simulink model "program_flight"  (R2022a)
settings: Solver=ode4  StartTime=0.0  StopTime=90  FixedStep=0.001  RelTol=1e-3
InitFcn:
  | BeforeSim
undefined symbols (not defined in the file or in its folder): d_ref, L_ref, S_ref
libraries: simulink_need_slupdate x10
settings Model: NumberOfSteps=10  PacingRate=0.010000  Creator=Hans  LastModifiedBy=24659
settings SolverCC: AlgebraicLoopSolver=TrustRegion
settings DataIOCC: ReturnWorkspaceOutputs=off
settings OptimizationCC: LifeSpan=inf
settings DebuggingCC: UnconnectedInputMsg=warning  UnconnectedOutputMsg=warning  UnconnectedLineMsg=warning  SFExecutionAtInitializationDiag=none  SFMachineParentedDataDiag=warning  ArithmeticOperatorsInVariantConditions=warning
settings HardwareCC: ProdBitPerSizeT=32  ProdBitPerPtrDiffT=32  ProdWordSize=32  ProdHWDeviceType=Specified
settings SFSimCC: SimUseLocalCustomCode=off  CustomCodeUndefinedFunction=UseInterfaceOnly
settings RTWCC: RTWUseLocalCustomCode=off
settings CodeAppCC: StateflowObjectComments=on

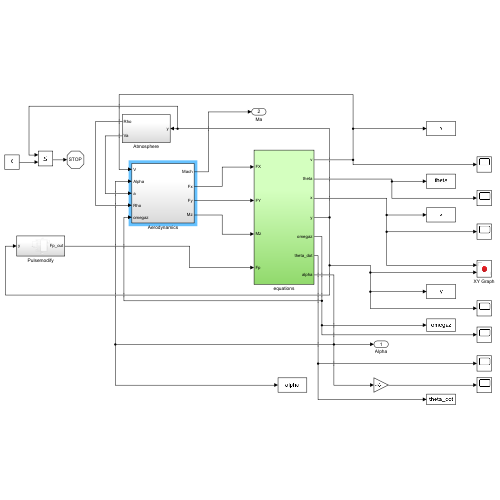
[thumbnail: Simulink's stored preview of the top-level diagram]
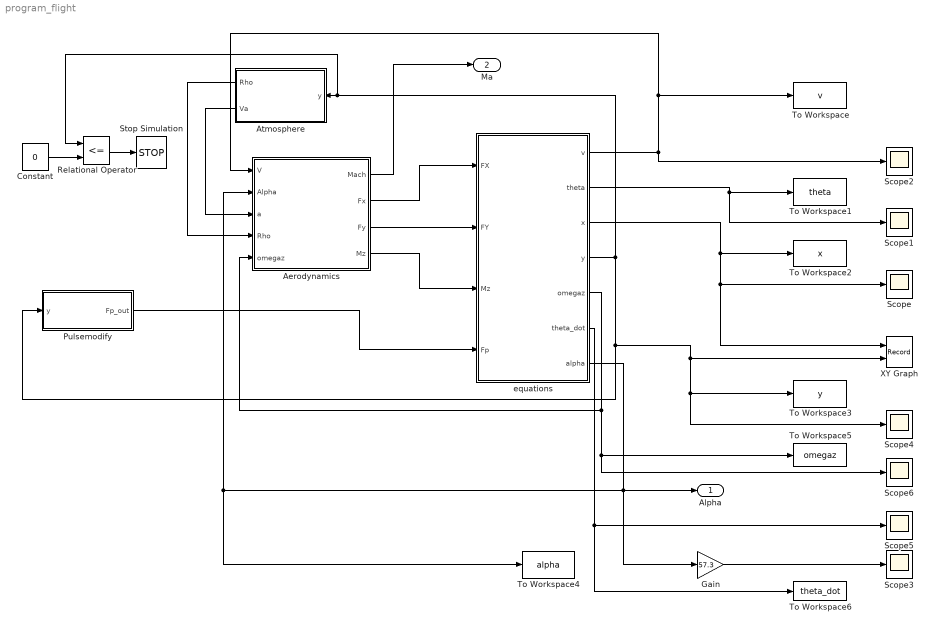
== system program_flight ==
  Aerodynamics : Subsystem
  Atmosphere : Subsystem
  Constant : Constant  Value=0
  Gain : Gain  Gain=57.3
  Pulsemodify : Subsystem
  Relational Operator : RelationalOperator  Operator=<=  OutDataTypeStr=boolean  RndMeth=Simplest  InputSameDT=off
  Scope{,1..6} (7 alike) : Scope
  Stop Simulation : Stop
  To Workspace : ToWorkspace  VariableName=v  SaveFormat=Timeseries  SampleTime=-1
  To Workspace1 : ToWorkspace  VariableName=theta  SaveFormat=Timeseries  SampleTime=-1
  To Workspace2 : ToWorkspace  VariableName=x  SaveFormat=Timeseries  SampleTime=-1
  To Workspace3 : ToWorkspace  VariableName=y  SaveFormat=Timeseries  SampleTime=-1
  To Workspace4 : ToWorkspace  VariableName=alpha  SaveFormat=Timeseries  SampleTime=-1
  To Workspace5 : ToWorkspace  VariableName=omegaz  SaveFormat=Timeseries  SampleTime=-1
  To Workspace6 : ToWorkspace  VariableName=theta_dot  SaveFormat=Timeseries  SampleTime=-1
  XY Graph : Record  FileSettingsInternal="{\"entries\":[{\"content\":{\"excelSettings\":{\"content\":{},\"type\":\"Streamout.ExcelSettings\"}},\"type\":\"Streamout.FileSettingStorage\",\"uuid\":\"457d8eac-be6b-48ff-b0a6-464f3e3e7ecd\"}],\"packageUris\":[\"http://schema.mathworks.com/mf0/streamout_blocks/R2020a\"],\"version\":\"1.0\"}"  Layout=[1 1]  SignalsInternal="{\"entries\":[{\"content\":{\"signals\":[{\"content\":{\"blockPath\":[\"program_flight/XY Graph\"],\"channel\":[],\"dimensions\":[1],\"domain\":\"program_flight/XY Graph\",\"lineColor\":\"#a2142f\",\"plots\":[1],\"port\":1,\"sid\":[\"\"],\"signalID\":2317,\"signalName\":\"equations:3\"},\"type\":\"RecordBlkView.Signal\",\"uuid\":\"4a28ca59-ac79-45de-aa29-5d33c689c1aa\"},{\"content\":{\"blockPath\":[\"program_flight/XY Graph\"],\"channel\":[],\"dimensions\":[1],\"domain\":\"program_flight/XY Graph\",\"lineColor\":\"#139fff\",\"plots\":[1],\"port\":2,\"sid\":[\"\"],\"signalID\":2321,\"signalName\":\"equations:4\"},\"type\":\"RecordBlkView.Signal\",\"uuid\":\"cb032477-1023-43de-a299-e45043520324\"}]},\"type\":\"RecordBlkView.InputSignals\",\"uuid\":\"09dcb611-f379-487a-ab87-7549ba248cf0\"}],\"packageUris\":[\"http://schema.mathworks.com/mf0/streamout_blocks/R2020a\"],\"version\":\"1.0\"}"  VisualizationBindings="{\"xyplotplugin\":{\"info\":[{\"series\":[{\"bindingParametersList\":[{\"parameter\":\"X-Axis\",\"signalID\":2317,\"signalName\":\"equations:3\"},{\"parameter\":\"Y-Axis\",\"signalID\":2321,\"signalName\":\"equations:4\"}],\"seriesID\":38071}],\"subplotID\":1}]}}"  CompatibilityTag=XY  st=-1
  equations : Subsystem
  Alpha : Outport
  Ma : Outport  Port=2
  wires:
  Gain/1 -> Scope3/1
  equations/4(y) -> Pulsemodify/1(y), To Workspace3/1, Scope4/1, XY Graph/2, Relational Operator/1, Atmosphere/1(y)
  equations/1(v) -> Aerodynamics/1(V), To Workspace/1, Scope2/1
  Aerodynamics/1(" Mach") -> Ma/1
  Aerodynamics/2(Fx) -> equations/1(FX)
  Atmosphere/1(Rho) -> Aerodynamics/4(Rho)
  Aerodynamics/3(Fy) -> equations/2(FY)
  Atmosphere/2(Va) -> Aerodynamics/3(a)
  equations/2(theta) -> Scope1/1, To Workspace1/1
  equations/3(x) -> XY Graph/1, Scope/1, To Workspace2/1
  equations/7(alpha) -> Gain/1, Aerodynamics/2(Alpha), To Workspace4/1, Alpha/1
  Aerodynamics/4(Mz) -> equations/3(Mz)
  equations/5(omegaz) -> Scope6/1, To Workspace5/1, Aerodynamics/5(omegaz)
  equations/6(theta_dot) -> To Workspace6/1, Scope5/1
  Constant/1 -> Relational Operator/2
  Relational Operator/1 -> Stop Simulation/1
  Pulsemodify/1(Fp_out) -> equations/4(Fp)

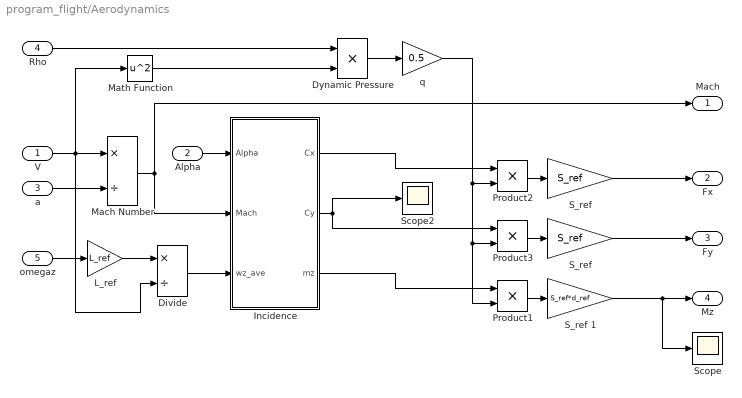
== system program_flight/Aerodynamics ==
  V : Inport
  Alpha : Inport  Port=2
  a : Inport  Port=3
  Rho : Inport  Port=4
  omegaz : Inport  Port=5
  Divide : Product  Inputs=*/
  Dynamic Pressure : Product  InputSameDT=on  SaturateOnIntegerOverflow=on  OutDataTypeStr=Inherit: Same as first input
  Incidence : Subsystem
  L_ref : Gain  Gain=L_ref  SaturateOnIntegerOverflow=on  OutDataTypeStr=Inherit: Same as input  ParamDataTypeStr=Inherit: Same as input
  Mach Number : Product  Inputs=*/  InputSameDT=on  SaturateOnIntegerOverflow=on  OutDataTypeStr=Inherit: Same as first input
  Math Function : Math  Operator=square  SignedPower=on
  Product1 : Product  InputSameDT=on  SaturateOnIntegerOverflow=on  OutDataTypeStr=Inherit: Same as first input
  Product2 : Product  InputSameDT=on  SaturateOnIntegerOverflow=on  OutDataTypeStr=Inherit: Same as first input
  Product3 : Product  InputSameDT=on  SaturateOnIntegerOverflow=on  OutDataTypeStr=Inherit: Same as first input
  S_ref : Gain  Gain=S_ref  SaturateOnIntegerOverflow=on  OutDataTypeStr=Inherit: Same as input  ParamDataTypeStr=Inherit: Same as input
  "S_ref " : Gain  Gain=S_ref  SaturateOnIntegerOverflow=on  OutDataTypeStr=Inherit: Same as input  ParamDataTypeStr=Inherit: Same as input
  S_ref 1 : Gain  Gain=S_ref*d_ref  SaturateOnIntegerOverflow=on  OutDataTypeStr=Inherit: Same as input  ParamDataTypeStr=Inherit: Same as input
  Scope : Scope
  Scope2 : Scope
  q : Gain  Gain=0.5  SaturateOnIntegerOverflow=on  OutDataTypeStr=Inherit: Same as input  ParamDataTypeStr=Inherit: Same as input
  " Mach" : Outport  InitialOutput=0
  Fx : Outport  Port=2  InitialOutput=[0]
  Fy : Outport  Port=3  InitialOutput=0
  Mz : Outport  Port=4
  wires:
  Incidence/2(Cy) -> Product3/1, Scope2/1
  Product3/1 -> "S_ref "/1
  S_ref/1 -> Fx/1
  "S_ref "/1 -> Fy/1
  Alpha/1 -> Incidence/1(Alpha)
  Product2/1 -> S_ref/1
  Mach Number/1 -> " Mach"/1, Incidence/2(Mach)
  a/1 -> Mach Number/2
  q/1 -> Product1/2, Product3/2, Product2/2
  Rho/1 -> Dynamic Pressure/1
  Dynamic Pressure/1 -> q/1
  Math Function/1 -> Dynamic Pressure/2
  Incidence/1(Cx) -> Product2/1
  Product1/1 -> S_ref 1/1
  S_ref 1/1 -> Scope/1, Mz/1
  Incidence/3(mz) -> Product1/1
  omegaz/1 -> L_ref/1
  L_ref/1 -> Divide/1
  Divide/1 -> Incidence/3(wz_ave)
  V/1 -> Divide/2, Math Function/1, Mach Number/1

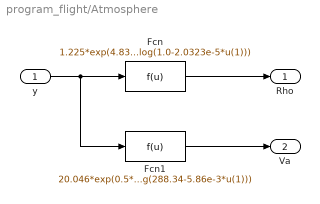
== system program_flight/Atmosphere ==
  y : Inport
  Fcn : Fcn  Expr=1.225*exp(4.83*log(1.0-2.0323e-5*u(1)))
  Fcn1 : Fcn  Expr=20.046*exp(0.5*log(288.34-5.86e-3*u(1)))
  Rho : Outport
  Va : Outport  Port=2
  wires:
  Fcn/1 -> Rho/1
  Fcn1/1 -> Va/1
  y/1 -> Fcn1/1, Fcn/1

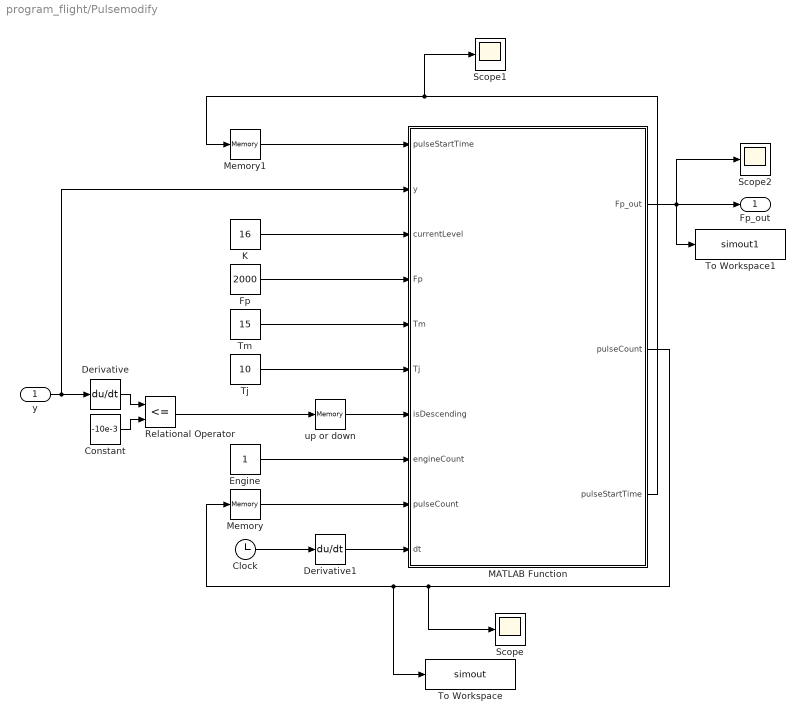
== system program_flight/Pulsemodify ==
  y : Inport
  Clock : Clock
  Constant : Constant  Value=-10e-3
  Derivative : Derivative
  Derivative1 : Derivative
  Engine : Constant
  Fp : Constant  Value=2000
  K : Constant  Value=16
  MATLAB Function : MATLAB Function  TreatAsAtomicUnit=on
  Memory : Memory
  Memory1 : Memory
  Relational Operator : RelationalOperator  Operator=<=  OutDataTypeStr=boolean  RndMeth=Simplest  InputSameDT=off
  Scope : Scope
  Scope1 : Scope
  Scope2 : Scope
  Tj : Constant  Value=10
  Tm : Constant  Value=15
  To Workspace : ToWorkspace  VariableName=simout  SaveFormat=Timeseries  SampleTime=-1
  To Workspace1 : ToWorkspace  VariableName=simout1  SaveFormat=Timeseries  SampleTime=-1
  up or down : Memory
  Fp_out : Outport
  wires:
  Fp/1 -> MATLAB Function/4(Fp)
  Tm/1 -> MATLAB Function/5(Tm)
  MATLAB Function/1(Fp_out) -> To Workspace1/1, Scope2/1, Fp_out/1
  y/1 -> MATLAB Function/2(y), Derivative/1
  Relational Operator/1 -> up or down/1
  up or down/1 -> MATLAB Function/7(isDescending)
  Derivative/1 -> Relational Operator/1
  Constant/1 -> Relational Operator/2
  K/1 -> MATLAB Function/3(currentLevel)
  Tj/1 -> MATLAB Function/6(Tj)
  Engine/1 -> MATLAB Function/8(engineCount)
  Memory1/1 -> MATLAB Function/1("pulseStartTime ")
  Memory/1 -> MATLAB Function/9("pulseCount ")
  MATLAB Function/2(pulseCount) -> Scope/1, To Workspace/1, Memory/1
  MATLAB Function/3(pulseStartTime) -> Scope1/1, Memory1/1
  Clock/1 -> Derivative1/1
  Derivative1/1 -> MATLAB Function/10(dt)

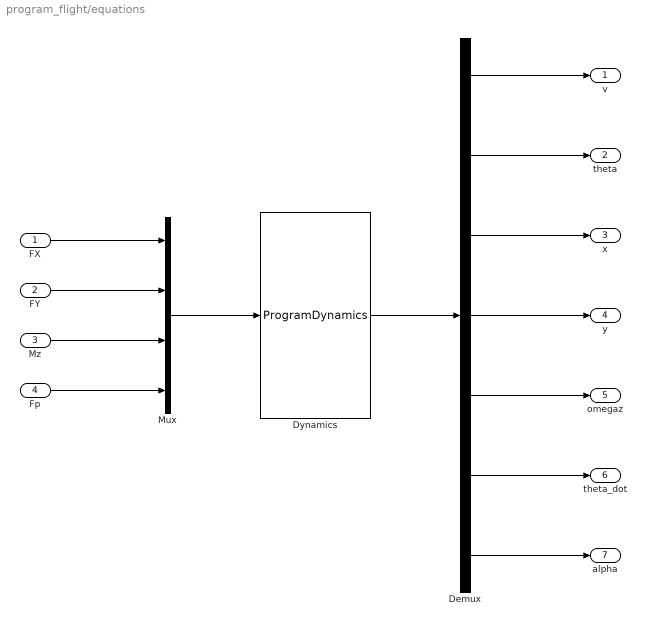
== system program_flight/equations ==
  FX : Inport
  FY : Inport  Port=2
  Mz : Inport  Port=3
  Fp : Inport  Port=4
  Demux : Demux  Outputs=7
  Dynamics : S-Function  FunctionName=ProgramDynamics  SFunctionDeploymentMode=off  EnableBusSupport=off
  Mux : Mux
  v : Outport
  theta : Outport  Port=2
  x : Outport  Port=3
  y : Outport  Port=4
  omegaz : Outport  Port=5
  theta_dot : Outport  Port=6
  alpha : Outport  Port=7
  wires:
  FX/1 -> Mux/1
  FY/1 -> Mux/2
  Mux/1 -> Dynamics/1
  Dynamics/1 -> Demux/1
  Demux/1 -> v/1
  Demux/2 -> theta/1
  Demux/3 -> x/1
  Demux/4 -> y/1
  Demux/7 -> alpha/1
  Demux/5 -> omegaz/1
  Mz/1 -> Mux/3
  Fp/1 -> Mux/4
  Demux/6 -> theta_dot/1

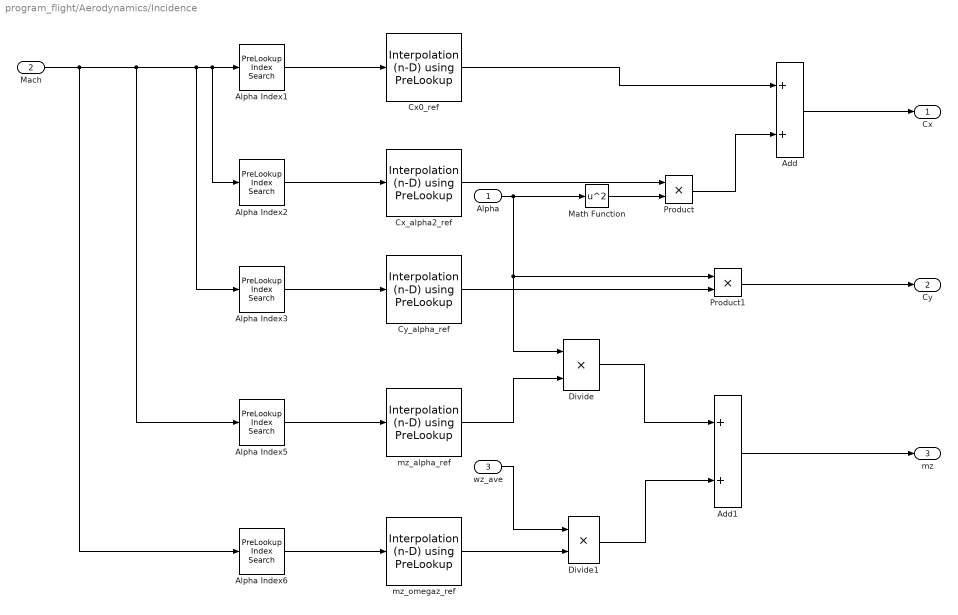
== system program_flight/Aerodynamics/Incidence ==
  Alpha : Inport
  Mach : Inport  Port=2
  wz_ave : Inport  Port=3
  Add : Sum
  Add1 : Sum
  Alpha Index{1..3,5..6} (5 alike) : simulink_need_slupdate/PreLookup Index Search  bpData=Mach_ref  searchMode=Binary Search  cacheBpFlag=on  outputFlag=off  IndexDataType=uint32  extrapMode=Linear Extrapolation  rangeErrorMode=None
      settings: SourceProductBaseCode=SL
  Cx0_ref : simulink_need_slupdate/Interpolation (n-D) using PreLookup  numDimsPopupSelect=1  explicitNumDims=2  table=Cx0_ref  interpMethod=Linear  extrapMethod=Linear  rangeErrorMode=None  NumSelectionDims=0
      settings: SourceProductBaseCode=SL
  Cx_alpha2_ref : simulink_need_slupdate/Interpolation (n-D) using PreLookup  numDimsPopupSelect=1  explicitNumDims=2  table=Cx_alpha2_ref  interpMethod=Linear  extrapMethod=Linear  rangeErrorMode=None  NumSelectionDims=0
      settings: SourceProductBaseCode=SL
  Cy_alpha_ref : simulink_need_slupdate/Interpolation (n-D) using PreLookup  numDimsPopupSelect=1  explicitNumDims=2  table=Cy_alpha_ref  interpMethod=Linear  extrapMethod=Linear  rangeErrorMode=None  NumSelectionDims=0
      settings: SourceProductBaseCode=SL
  Divide : Product
  Divide1 : Product
  Math Function : Math  Operator=square  SignedPower=on
  Product : Product
  Product1 : Product
  mz_alpha_ref : simulink_need_slupdate/Interpolation (n-D) using PreLookup  numDimsPopupSelect=1  explicitNumDims=2  table=mz_alpha_ref  interpMethod=Linear  extrapMethod=Linear  rangeErrorMode=None  NumSelectionDims=0
      settings: SourceProductBaseCode=SL
  mz_omegaz_ref : simulink_need_slupdate/Interpolation (n-D) using PreLookup  numDimsPopupSelect=1  explicitNumDims=2  table=mz_omegaz_ref  interpMethod=Linear  extrapMethod=Linear  rangeErrorMode=None  NumSelectionDims=0
      settings: SourceProductBaseCode=SL
  Cx : Outport  InitialOutput=0
  Cy : Outport  Port=2  InitialOutput=0
  mz : Outport  Port=3
  wires:
  Alpha Index1/1 -> Cx0_ref/1
  Alpha Index2/1 -> Cx_alpha2_ref/1
  Alpha Index3/1 -> Cy_alpha_ref/1
  Alpha Index5/1 -> mz_alpha_ref/1
  Alpha Index6/1 -> mz_omegaz_ref/1
  Mach/1 -> Alpha Index6/1, Alpha Index5/1, Alpha Index3/1, Alpha Index2/1, Alpha Index1/1
  Cx_alpha2_ref/1 -> Product/1
  Math Function/1 -> Product/2
  Cx0_ref/1 -> Add/1
  Product/1 -> Add/2
  Add/1 -> Cx/1
  Cy_alpha_ref/1 -> Product1/2
  Divide/1 -> Add1/1
  Add1/1 -> mz/1
  Product1/1 -> Cy/1
  mz_alpha_ref/1 -> Divide/2
  Alpha/1 -> Math Function/1, Divide/1, Product1/1
  mz_omegaz_ref/1 -> Divide1/2
  wz_ave/1 -> Divide1/1
  Divide1/1 -> Add1/2

== matlab function program_flight/Pulsemodify/MATLAB Function ==
  data: pulseStartTime input; y input; currentLevel input; Fp input; Tm input; Tj input; isDescending input; engineCount input; pulseCount input; Fp_out output; pulseCount output; pulseStartTime output; dt input
function [Fp_out, pulseCount, pulseStartTime] = computeImpulseForce(pulseStartTime, y, currentLevel, Fp, Tm, Tj, isDescending, engineCount, pulseCount, dt)
Fp_out = 0;

% 如果飞行器在下降，并且高度小于2000m
if isDescending && y <= 2000
    % 计算当前脉冲级数
    if pulseCount < currentLevel * engineCount
        % 判断当前时间是否在脉冲持续时间内
        if pulseStartTime < Tm
            Fp_out = Fp;
            pulseStartTime = pulseStartTime + dt;  % 更新脉冲开始时间
        % 判断当前时间是否在脉冲间隔时间内
        elseif pulseStartTime < Tm + Tj
            Fp_out = 0;
            pulseStartTime = pulseStartTime + dt;  % 更新脉冲开始时间
        % 脉冲间隔时间结束，开始新的脉冲
        else
            pulseStartTime = 0;
            pulseCount = pulseCount + 1;
        end
    end
end
end
